simulink model "Fzg_Beschleunigen_Rueckschaltung"  (R2013a)
settings: Solver=ode45  StartTime=0.0  StopTime=20  FixedStep=0.001  RelTol=1e-3
PostLoadFcn:
  | , if any(exist('dsrtsu_mdlpostloadfcn', 'file') == [2, 3, 6]), try dsrtsu_mdlpostloadfcn('Execute', bdroot); catch fprintf('Error in PostLoadFcn (dsrtsu_mdlpostloadfcn) for model "%s":\n %s\n', bdroot, lasterr); end, end,
values from neighbouring files (symbols this model uses):
  A = 1.7    [Parameter_Beschleunigen_Rueckschaltung.m]
  c_W = 0.32    [Parameter_Beschleunigen_Rueckschaltung.m]
  eta = 0.9    [Parameter_Beschleunigen_Rueckschaltung.m]
  F_R = 160    [Parameter_Beschleunigen_Rueckschaltung.m]
  i_A = 4.06    [Parameter_Beschleunigen_Rueckschaltung.m]
  i_G4 = 2.1    [Parameter_Beschleunigen_Rueckschaltung.m]
  i_G5 = 1.3    [Parameter_Beschleunigen_Rueckschaltung.m]
  m = 1600    [Parameter_Beschleunigen_Rueckschaltung.m]
  r_R = 0.291    [Parameter_Beschleunigen_Rueckschaltung.m]
  rho = 1.2    [Parameter_Beschleunigen_Rueckschaltung.m]
  v_0 = 60/3.6    (= 16.6666666667)    [Parameter_Beschleunigen_Rueckschaltung.m]
  v_max = r_R * omega_Rad_max    (= 37.5288777584)    [Parameter_Beschleunigen_Rueckschaltung.m]
  v_max_4 = r_R * omega_Rad_max_4    (= 23.2321624219)    [Parameter_Beschleunigen_Rueckschaltung.m]
libraries: simulink x1
settings Model: DSRTSU_INTERNAL_RTI_VER=430  DSRTSU_INTERNAL_RTI_TYPE=rti1401  DSRTSU_INTERNAL_RTIFPGA=20  BufferReuse=off  Creator=schiele  LastModifiedBy=schiele
settings OptimizationCC: BlockReduction=off  OptimizeBlockIOStorage=off  BufferReuse=off  ExpressionFolding=off  LocalBlockOutputs=off
settings HardwareCC: ProdIntDivRoundTo=Zero  ProdEndianess=BigEndian  ProdHWDeviceType=Generic->Custom  TargetIntDivRoundTo=Zero  TargetEndianess=BigEndian  TargetHWDeviceType=Generic->Custom
settings RTWCC: SystemTargetFile=rti1401.tlc  MakeCommand=make_rti  TemplateMakefile=rti1401.tmf  Description=dSPACE DS1401 Hardware Platform  ProcessScript=rti1401_make_rtw_hook
settings STFCustomTargetCC: ParMdlRefBuildCompliant=on  GeneratePreprocessorConditionals=Disable all  MatFileLogging=on  GRTInterface=on  SystemTargetFile=rti1401.tlc
settings GRTTargetCC: CompOptLevelCompliant=off  ConcurrentExecutionCompliant=off  CombineOutputUpdateFcns=off  GRTInterface=on  ExtModeMexFile=noextcomm

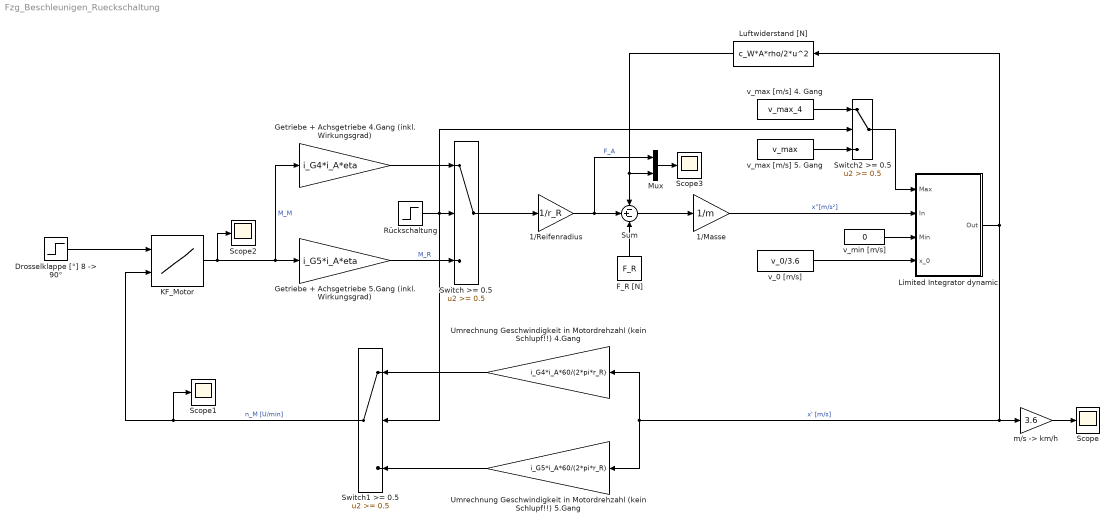
== system Fzg_Beschleunigen_Rueckschaltung ==
  1/Masse : Gain  Gain=1/m
  1/Reifenradius : Gain  Gain=1/r_R
  "Drosselklappe [°] 8 -> 90°" : Step  Time=5  Before=8  After=90  SampleTime=0
  F_R [N] : Constant  Value=F_R
  "Getriebe + Achsgetriebe 4.Gang (inkl. Wirkungsgrad) " : Gain  Gain=i_G4*i_A*eta
  Getriebe + Achsgetriebe 5.Gang (inkl. Wirkungsgrad) : Gain  Gain=i_G5*i_A*eta
  KF_Motor : Lookup_n-D  BreakpointsForDimension1=KF_Motor(2:end,1)  BreakpointsForDimension2=KF_Motor(1,2:end)  Table=KF_Motor(2:end,2:end)  RndMeth=Simplest  InputSameDT=on
      settings: OpenFcn=kf_plot
  Limited Integrator dynamic : Subsystem
  Luftwiderstand [N] : Fcn  Expr=c_W*A*rho/2*u^2
  Mux : Mux  Inputs=2
  Rückschaltung : Step  Time=5  SampleTime=0
  Scope{,1..3} (4 alike) : Scope
      Scope settings: SaveName=Erg_v
      Scope1 settings: SaveName=Erg_n
      Scope2 settings: SaveName=Erg_M
      Scope3 settings: SaveName=Erg_F
  Sum : Sum  Inputs=-+-
  Switch >= 0.5 : Switch  Threshold=0.5
  Switch1 >= 0.5 : Switch  Threshold=0.5
  Switch2 >= 0.5 : Switch  Threshold=0.5
  Umrechnung Geschwindigkeit in Motordrehzahl (kein Schlupf!!) 4.Gang : Gain  Gain=i_G4*i_A*60/(2*pi*r_R)
  Umrechnung Geschwindigkeit in Motordrehzahl (kein Schlupf!!) 5.Gang : Gain  Gain=i_G5*i_A*60/(2*pi*r_R)
  "m/s -> km/h" : Gain  Gain=3.6
  v_0 [m/s] : Constant  Value=v_0/3.6
  v_max [m/s] 4. Gang : Constant  Value=v_max_4
  v_max [m/s] 5. Gang : Constant  Value=v_max
  v_min [m/s] : Constant  Value=0
  wires:
  "Drosselklappe [°] 8 -> 90°"/1 -> KF_Motor/1
  KF_Motor/1 -> "Getriebe + Achsgetriebe 4.Gang (inkl. Wirkungsgrad) "/1, Getriebe + Achsgetriebe 5.Gang (inkl. Wirkungsgrad)/1, Scope2/1  "M_M"
  1/Reifenradius/1 -> Mux/1, Sum/2  "F_A"
  F_R [N]/1 -> Sum/3
  Luftwiderstand [N]/1 -> Mux/2, Sum/1
  Sum/1 -> 1/Masse/1
  1/Masse/1 -> Limited Integrator dynamic/2(In)  "x''[m/s²]"
  v_0 [m/s]/1 -> Limited Integrator dynamic/4(x_0)
  Limited Integrator dynamic/1(Out) -> Luftwiderstand [N]/1, Umrechnung Geschwindigkeit in Motordrehzahl (kein Schlupf!!) 5.Gang/1, Umrechnung Geschwindigkeit in Motordrehzahl (kein Schlupf!!) 4.Gang/1, "m/s -> km/h"/1  "x' [m/s]"
  Switch1 >= 0.5/1 -> Scope1/1, KF_Motor/2  "n_M [U/min]"
  "m/s -> km/h"/1 -> Scope/1
  Mux/1 -> Scope3/1
  Getriebe + Achsgetriebe 5.Gang (inkl. Wirkungsgrad)/1 -> Switch >= 0.5/3  "M_R"
  "Getriebe + Achsgetriebe 4.Gang (inkl. Wirkungsgrad) "/1 -> Switch >= 0.5/1
  Switch >= 0.5/1 -> 1/Reifenradius/1
  Rückschaltung/1 -> Switch2 >= 0.5/2, Switch1 >= 0.5/2, Switch >= 0.5/2
  Umrechnung Geschwindigkeit in Motordrehzahl (kein Schlupf!!) 4.Gang/1 -> Switch1 >= 0.5/1
  Umrechnung Geschwindigkeit in Motordrehzahl (kein Schlupf!!) 5.Gang/1 -> Switch1 >= 0.5/3
  v_min [m/s]/1 -> Limited Integrator dynamic/3(Min)
  Switch2 >= 0.5/1 -> Limited Integrator dynamic/1(Max)
  v_max [m/s] 5. Gang/1 -> Switch2 >= 0.5/3
  v_max [m/s] 4. Gang/1 -> Switch2 >= 0.5/1

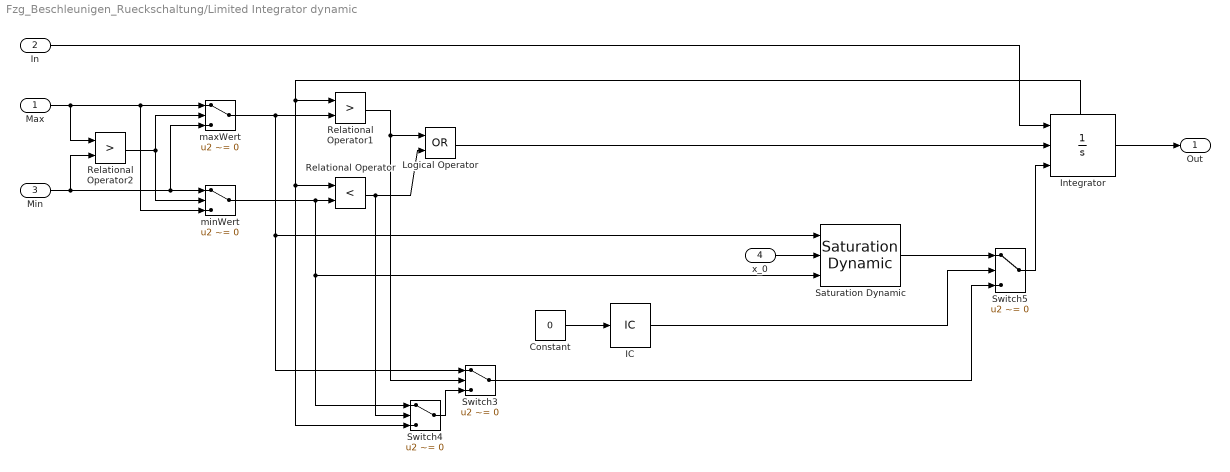
== system Fzg_Beschleunigen_Rueckschaltung/Limited Integrator dynamic ==
  Max : Inport
  In : Inport  Port=2
  Min : Inport  Port=3
  x_0 : Inport  Port=4
  Constant : Constant  Value=0
  IC : InitialCondition
  Integrator : Integrator  ExternalReset=level  InitialConditionSource=external  ShowStatePort=on
  Logical Operator : Logic  Operator=OR  AllPortsSameDT=off  OutDataTypeStr=boolean
  Relational Operator : RelationalOperator  Operator=<  OutDataTypeStr=boolean
  Relational Operator1 : RelationalOperator  Operator=>  OutDataTypeStr=boolean
  Relational Operator2 : RelationalOperator  Operator=>  OutDataTypeStr=boolean
  Saturation Dynamic : simulink/Discontinuities/Saturation Dynamic  OutMin=[]  OutMax=[]  OutDataTypeStr=Inherit: Same as second input  OutDataType=fixdt(1, 16)  OutScaling=2^-10  DoSatur=off
  Switch3 : Switch  Criteria=u2 ~= 0
  Switch4 : Switch  Criteria=u2 ~= 0
  Switch5 : Switch  Criteria=u2 ~= 0
  maxWert : Switch  Criteria=u2 ~= 0
  minWert : Switch  Criteria=u2 ~= 0
  Out : Outport
  wires:
  Integrator/1 -> Out/1
  maxWert/1 -> Relational Operator1/2, Switch3/1, Saturation Dynamic/1
  minWert/1 -> Relational Operator/2, Switch4/1, Saturation Dynamic/3
  Relational Operator1/1 -> Logical Operator/1, Switch3/2
  Relational Operator/1 -> Logical Operator/2, Switch4/2
  Max/1 -> minWert/3, maxWert/1, Relational Operator2/1
  Min/1 -> minWert/1, maxWert/3, Relational Operator2/2
  Relational Operator2/1 -> maxWert/2, minWert/2
  In/1 -> Integrator/1
  Integrator/State -> Relational Operator1/1, Relational Operator/1, Switch4/3
  Switch4/1 -> Switch3/3
  Logical Operator/1 -> Integrator/2
  Switch5/1 -> Integrator/3
  x_0/1 -> Saturation Dynamic/2
  Constant/1 -> IC/1
  Saturation Dynamic/1 -> Switch5/1
  IC/1 -> Switch5/2
  Switch3/1 -> Switch5/3
